simulink model "DLS_ex2"  (R2025b)
settings: Solver=VariableStepAuto  StartTime=0  StopTime=200000  FixedStep=0.5  MaxStep=200  MinStep=0.1  RelTol=.0001
model workspace (MATLAB code in the model file):
  Temp_Ambient = 295.15
  Temp_Environment = 295.15
  Time_Warmup = 200000
  Density_Copper = 8960/1000000000    (= 8.96e-06)
  Density_G10 = 1800/1000000000    (= 1.8e-06)
  Density_Stainless_Steel = 7930/1000000000    (= 7.93e-06)
  Density_Aluminium = 2700/1000000000    (= 2.7e-06)
  Density_Titanium = 4500/1000000000    (= 4.5e-06)
  Density_Aluminium_Nitride = 3300/1000000000    (= 3.3e-06)
  Density_Invar = 8050/1000000000    (= 8.05e-06)
  SHC_Copper = 386
  SHC_G10 = 500
  SHC_Stainless_Steel = 500
  SHC_Aluminium = 900
  SHC_Titanium = 528
  SHC_Aluminium_Nitride = 820
  SHC_Phosphor_Bronze = 377
  SHC_Invar = 515
  K_B1_LB = 2.83489E-08    (= 2.83489e-08)
  K_B1_RE = 1.13396E-08    (= 1.13396e-08)
  K_B1_UB = 5.66944E-09    (= 5.66944e-09)
  K_B2_LB = 5.15455E-10    (= 5.15455e-10)
  K_B2_RE = 2.3625E-10    (= 2.3625e-10)
  K_B2_UB = 9.61017E-11    (= 9.61017e-11)
  K_B3_LB = 5.15455E-09    (= 5.15455e-09)
  K_B3_RE = 2.3625E-09    (= 2.3625e-09)
  K_B3_UB = 9.61017E-10    (= 9.61017e-10)
  K_B4_LB = 5.15455E-09    (= 5.15455e-09)
  K_B4_RE = 2.3625E-09    (= 2.3625e-09)
  K_B4_UB = 9.61017E-10    (= 9.61017e-10)
  K_B5_LB = 5.15455E-09    (= 5.15455e-09)
  K_B5_RE = 2.3625E-09    (= 2.3625e-09)
  K_B5_UB = 9.61017E-10    (= 9.61017e-10)
  K_B6_LB = 5.15455E-09    (= 5.15455e-09)
  K_B6_RE = 2.3625E-09    (= 2.3625e-09)
  K_B6_UB = 9.61017E-10    (= 9.61017e-10)
  K_B7_LB = 5.67E-09    (= 5.67e-09)
  K_B7_RE = 2.8E-09    (= 2.8e-09)
  K_B7_UB = 1.11176E-09    (= 1.11176e-09)
  K_B8_LB = 5.67E-09    (= 5.67e-09)
  K_B8_RE = 2.8E-09    (= 2.8e-09)
  K_B8_UB = 1.11176E-09    (= 1.11176e-09)
  K_B9_LB = 2.835E-08    (= 2.835e-08)
  K_B9_RE = 1.08E-08    (= 1.08e-08)
  K_B9_UB = 5.15455E-09    (= 5.15455e-09)
  K_B10_LB = 4.78193E-09    (= 4.78193e-09)
  K_B10_RE = 8.95937E-10    (= 8.95937e-10)
  K_B10_UB = 2.20909E-09    (= 2.20909e-09)
  K_B13_LB = 3.54375E-09    (= 3.54375e-09)
  K_B13_RE = 1.73571E-09    (= 1.73571e-09)
  K_B13_UB = 6.85887E-10    (= 6.85887e-10)
  K_B14_LB = 2.98421E-09    (= 2.98421e-09)
  K_B14_RE = 1.45385E-09    (= 1.45385e-09)
  K_B14_UB = 5.72727E-10    (= 5.72727e-10)
  K_B15_LB = 4.05E-10    (= 4.05e-10)
  K_B15_RE = 1.95517E-10    (= 1.95517e-10)
  K_B15_UB = 5.72727E-11    (= 5.72727e-11)
  K_B16_LB = 4.05E-09    (= 4.05e-09)
  K_B16_RE = 1.95517E-09    (= 1.95517e-09)
  K_B16_UB = 5.72727E-10    (= 5.72727e-10)
  K_B17_LB = 2.83458E-09    (= 2.83458e-09)
  K_B17_RE = 1.13386E-09    (= 1.13386e-09)
  K_B17_UB = 5.66908E-10    (= 5.66908e-10)
  K_B18_LB = 2.83458E-09    (= 2.83458e-09)
  K_B18_RE = 1.13386E-09    (= 1.13386e-09)
  K_B18_UB = 5.66908E-10    (= 5.66908e-10)
  K_B19_LB = 2.83458E-09    (= 2.83458e-09)
  K_B19_RE = 1.13386E-09    (= 1.13386e-09)
  K_B19_UB = 5.66908E-10    (= 5.66908e-10)
  K_B20_LB = 5.15455E-10    (= 5.15455e-10)
  K_B20_RE = 2.3625E-10    (= 2.3625e-10)
  K_B20_UB = 9.61017E-11    (= 9.61017e-11)
  K_B21_LB = 9.45E-09    (= 9.45e-09)
  K_B21_RE = 4.05E-09    (= 4.05e-09)
  K_B21_UB = 9.61017E-10    (= 9.61017e-10)
  K_B22_LB = 4.78193E-09    (= 4.78193e-09)
  K_B22_RE = 2.20909E-09    (= 2.20909e-09)
  K_B22_UB = 8.95937E-10    (= 8.95937e-10)
  K_B23_LB = 5.15455E-09    (= 5.15455e-09)
  K_B23_RE = 2.3625E-09    (= 2.3625e-09)
  K_B23_UB = 9.61017E-10    (= 9.61017e-10)
  K_B25_LB = 2.98421E-09    (= 2.98421e-09)
  K_B25_RE = 1.45385E-09    (= 1.45385e-09)
  K_B25_UB = 5.72727E-10    (= 5.72727e-10)
  K_B1 = K_B1_RE    (= 1.13396e-08)
  K_B2 = K_B2_RE    (= 2.3625e-10)
  K_B3 = K_B3_RE    (= 2.3625e-09)
  K_B4 = K_B4_RE    (= 2.3625e-09)
  K_B5 = K_B5_RE    (= 2.3625e-09)
  K_B6 = K_B6_RE    (= 2.3625e-09)
  K_B7 = K_B7_RE    (= 2.8e-09)
  K_B8 = K_B8_RE    (= 2.8e-09)
  K_B9 = K_B9_RE    (= 1.08e-08)
  K_B10 = K_B10_RE    (= 8.95937e-10)
  K_B13 = K_B13_RE    (= 1.73571e-09)
  K_B14 = K_B14_RE    (= 1.45385e-09)
  K_B15 = K_B15_RE    (= 1.95517e-10)
  K_B16 = K_B16_RE    (= 1.95517e-09)
  K_B17 = K_B17_RE    (= 1.13386e-09)
  K_B18 = K_B18_RE    (= 1.13386e-09)
  K_B19 = K_B19_RE    (= 1.13386e-09)
  K_B20 = K_B20_RE    (= 2.3625e-10)
  K_B21 = K_B21_RE    (= 4.05e-09)
  K_B22 = K_B22_RE    (= 2.20909e-09)
  K_B23 = K_B23_RE    (= 2.3625e-09)
  K_B25 = K_B25_RE    (= 1.45385e-09)
  Area_B1 = 100000
  Area_B2 = 30000
  Area_B3 = 450
  Area_B4 = 613
  Area_B5 = 4410
  Area_B6 = 1590
  Area_B7 = 120
  Area_B8 = 50
  Area_B9 = 140
  Area_B10 = 100
  Area_B13 = 9990
  Area_B14 = 7710
  Area_B15 = 10000
  Area_B16 = 2000
  Area_B17 = 70015
  Area_B18 = 16000
  Area_B19 = 320000
  Area_B20 = 70000
  Area_B21 = 4000
  Area_B22 = 4900
  Area_B23 = 9155
  Area_B25 = 4072
  xt = linspace(5,295,2000)
  x_restemp = [4	10	20	30	40	50	60	70	80	90	100	110	120	130	140	150	160	170	180	190	200	210	220	230	240	250	260	273	280	293	300]
  y_res_A1_LB = [1.852847068	0.77281194	0.49125288	0.555353451	0.801331659	1.184325573	1.60557094	1.971748902	2.248473254	2.443766462	2.578413714	2.67150152	2.736985932	2.784247759	2.819401592	2.846406384	2.867837824	2.885389229	2.900188421	2.912997223	2.924337653	2.934572526	2.943957542	2.95267538	2.960858317	2.96860341	2.975982825	2.985117154	2.989849299	2.998335893	3.002758516]
  res_A1_LB = (akima(x_restemp,y_res_A1_LB,xt))'
  y_res_A1_RE = [1.558179157	0.649907636	0.413126378	0.467032702	0.673891715	0.995976115	1.350228639	1.658171414	1.890886853	2.055121565	2.168355165	2.246638732	2.301708818	2.34145435	2.371017486	2.393727565	2.411750652	2.426510766	2.438956365	2.449728117	2.459265019	2.467872188	2.475764655	2.48309605	2.489977612	2.496490963	2.502696791	2.51037844	2.514358008	2.521494934	2.525214205]
  res_A1_RE = (akima(x_restemp,y_res_A1_RE,xt))'
  y_res_A1_UB = [1.383495056	0.577047894	0.366811672	0.414674674	0.59834317	0.884319383	1.198857421	1.472277397	1.67890361	1.824726324	1.925265549	1.994772914	2.043669212	2.078958958	2.105207835	2.125371936	2.141374494	2.154479883	2.165530233	2.175094387	2.183562128	2.191204365	2.198212025	2.204721514	2.210831598	2.216614751	2.222124857	2.228945334	2.23247876	2.238815581	2.242117892]
  res_A1_UB = (akima(x_restemp,y_res_A1_UB,xt))'
  y_res_A2_LB = [0.466691844	0.194654505	0.123735907	0.139881445	0.201838001	0.298305832	0.40440837	0.496640627	0.566341468	0.615531576	0.649446288	0.67289308	0.689387178	0.701291403	0.710145888	0.716947808	0.722345921	0.726766738	0.730494332	0.73372059	0.736576998	0.73915494	0.741518821	0.743714655	0.745775758	0.747726578	0.749585292	0.751886031	0.753077956	0.755215544	0.756329506]
  res_A2_LB = (akima(x_restemp,y_res_A2_LB,xt))'
  y_res_A2_RE = [0.422241188	0.17611439	0.111950524	0.12655826	0.182613685	0.269893315	0.365889982	0.449337462	0.512399558	0.556904491	0.587588954	0.608802526	0.623725623	0.634496015	0.642507144	0.648661206	0.653545169	0.657544919	0.660917474	0.663836444	0.666420789	0.668753191	0.670891922	0.67287861	0.674743402	0.676508414	0.678190092	0.680271694	0.681350092	0.683284083	0.684291945]
  res_A2_RE = (akima(x_restemp,y_res_A2_RE,xt))'
  y_res_A2_UB = [0.385689258	0.160868789	0.102259362	0.115602558	0.166805463	0.246529603	0.334216178	0.410439904	0.468042936	0.508695235	0.536723452	0.55610064	0.569731897	0.579569934	0.586887568	0.592508894	0.59697007	0.600623576	0.603704181	0.606370465	0.608731093	0.610861588	0.612815176	0.614629884	0.616333247	0.617945468	0.619481569	0.621382974	0.622368019	0.624134591	0.625055206]
  res_A2_UB = (akima(x_restemp,y_res_A2_UB,xt))'
  y_res_A3_LB = [0.466691844	0.194654505	0.123735907	0.139881445	0.201838001	0.298305832	0.40440837	0.496640627	0.566341468	0.615531576	0.649446288	0.67289308	0.689387178	0.701291403	0.710145888	0.716947808	0.722345921	0.726766738	0.730494332	0.73372059	0.736576998	0.73915494	0.741518821	0.743714655	0.745775758	0.747726578	0.749585292	0.751886031	0.753077956	0.755215544	0.756329506]
  res_A3_LB = (akima(x_restemp,y_res_A3_LB,xt))'
  y_res_A3_RE = [0.422241188	0.17611439	0.111950524	0.12655826	0.182613685	0.269893315	0.365889982	0.449337462	0.512399558	0.556904491	0.587588954	0.608802526	0.623725623	0.634496015	0.642507144	0.648661206	0.653545169	0.657544919	0.660917474	0.663836444	0.666420789	0.668753191	0.670891922	0.67287861	0.674743402	0.676508414	0.678190092	0.680271694	0.681350092	0.683284083	0.684291945]
  res_A3_RE = (akima(x_restemp,y_res_A3_RE,xt))'
  y_res_A3_UB = [0.385689258	0.160868789	0.102259362	0.115602558	0.166805463	0.246529603	0.334216178	0.410439904	0.468042936	0.508695235	0.536723452	0.55610064	0.569731897	0.579569934	0.586887568	0.592508894	0.59697007	0.600623576	0.603704181	0.606370465	0.608731093	0.610861588	0.612815176	0.614629884	0.616333247	0.617945468	0.619481569	0.621382974	0.622368019	0.624134591	0.625055206]
  res_A3_UB = (akima(x_restemp,y_res_A3_UB,xt))'
  y_res_A4_LB = [1.668225823	0.695807472	0.442303498	0.500016965	0.721485431	1.066317096	1.445588764	1.77528005	2.024431055	2.200264872	2.321495613	2.405307971	2.464267391	2.506819958	2.538470996	2.562784978	2.582080948	2.597883497	2.611208069	2.622740577	2.632951025	2.642166076	2.650615951	2.658465127	2.665832701	2.672806057	2.679450173	2.68767434	2.691934966	2.699575939	2.703557883]
  res_A4_LB = (akima(x_restemp,y_res_A4_LB,xt))'
  y_res_A4_RE = [1.40291919	0.585149589	0.371961671	0.420496665	0.606743849	0.896735139	1.215689261	1.492948026	1.70247525	1.8503453	1.952296086	2.022779328	2.072362125	2.108147336	2.134764744	2.155211947	2.171439179	2.184728567	2.195934063	2.205632496	2.214219123	2.221968657	2.229074704	2.235675585	2.241871455	2.247735802	2.253323269	2.260239505	2.263822541	2.27024833	2.273597005]
  res_A4_RE = (akima(x_restemp,y_res_A4_RE,xt))'
  y_res_A4_UB = [1.245640948	0.519549732	0.330261851	0.373355692	0.538723106	0.796204099	1.079400963	1.325576846	1.511614426	1.642907084	1.733428387	1.796009905	1.840034081	1.87180749	1.895440878	1.913595789	1.928003821	1.939803364	1.949752636	1.958363799	1.965987798	1.972868548	1.979177952	1.985038822	1.990540086	1.995746994	2.000708063	2.006848934	2.010030283	2.015735691	2.018708954]
  res_A4_UB = (akima(x_restemp,y_res_A4_UB,xt))'
  y_res_A5_LB = [1.101209878	0.459308357	0.291968254	0.330065398	0.476258593	0.703884871	0.954245285	1.171877272	1.336343943	1.452413323	1.532438753	1.587763994	1.626683603	1.65477291	1.675666025	1.691715889	1.704453321	1.714884717	1.723680379	1.731293084	1.738033087	1.744116019	1.749693853	1.75487516	1.759738557	1.764341728	1.768727565	1.774156407	1.776968881	1.782012752	1.784641267]
  res_A5_LB = (akima(x_restemp,y_res_A5_LB,xt))'
  y_res_A5_RE = [0.951197386	0.396739002	0.252194832	0.285102187	0.41138019	0.607998042	0.824253069	1.012238103	1.154300276	1.254558086	1.323682039	1.37147059	1.405088369	1.429351206	1.447398153	1.461261622	1.472263895	1.481274272	1.488871744	1.495447407	1.501269252	1.506523536	1.511341528	1.515817011	1.520017891	1.523993994	1.527782369	1.532471667	1.534901011	1.53925778	1.541528225]
  res_A5_RE = (akima(x_restemp,y_res_A5_RE,xt))'
  y_res_A5_UB = [0.837873198	0.34947213	0.222148729	0.251135552	0.36236899	0.535562094	0.726052831	0.891641619	1.016778724	1.105091973	1.165980605	1.208075702	1.23768831	1.25906051	1.274957372	1.287169169	1.296860648	1.304797543	1.311489863	1.317282112	1.322410351	1.327038648	1.331282632	1.335224913	1.338925306	1.342427703	1.345764737	1.349895359	1.352035275	1.355872985	1.357872932]
  res_A5_UB = (akima(x_restemp,y_res_A5_UB,xt))'
  y_res_A6_LB = [0.466691844	0.194654505	0.123735907	0.139881445	0.201838001	0.298305832	0.40440837	0.496640627	0.566341468	0.615531576	0.649446288	0.67289308	0.689387178	0.701291403	0.710145888	0.716947808	0.722345921	0.726766738	0.730494332	0.73372059	0.736576998	0.73915494	0.741518821	0.743714655	0.745775758	0.747726578	0.749585292	0.751886031	0.753077956	0.755215544	0.756329506]
  res_A6_LB = (akima(x_restemp,y_res_A6_LB,xt))'
  y_res_A6_RE = [0.422241188	0.17611439	0.111950524	0.12655826	0.182613685	0.269893315	0.365889982	0.449337462	0.512399558	0.556904491	0.587588954	0.608802526	0.623725623	0.634496015	0.642507144	0.648661206	0.653545169	0.657544919	0.660917474	0.663836444	0.666420789	0.668753191	0.670891922	0.67287861	0.674743402	0.676508414	0.678190092	0.680271694	0.681350092	0.683284083	0.684291945]
  res_A6_RE = (akima(x_restemp,y_res_A6_RE,xt))'
  y_res_A6_UB = [0.385689258	0.160868789	0.102259362	0.115602558	0.166805463	0.246529603	0.334216178	0.410439904	0.468042936	0.508695235	0.536723452	0.55610064	0.569731897	0.579569934	0.586887568	0.592508894	0.59697007	0.600623576	0.603704181	0.606370465	0.608731093	0.610861588	0.612815176	0.614629884	0.616333247	0.617945468	0.619481569	0.621382974	0.622368019	0.624134591	0.625055206]
  res_A6_UB = (akima(x_restemp,y_res_A6_UB,xt))'
  y_res_A7_LB = [0.466691844	0.194654505	0.123735907	0.139881445	0.201838001	0.298305832	0.40440837	0.496640627	0.566341468	0.615531576	0.649446288	0.67289308	0.689387178	0.701291403	0.710145888	0.716947808	0.722345921	0.726766738	0.730494332	0.73372059	0.736576998	0.73915494	0.741518821	0.743714655	0.745775758	0.747726578	0.749585292	0.751886031	0.753077956	0.755215544	0.756329506]
  res_A7_LB = (akima(x_restemp,y_res_A7_LB,xt))'
  y_res_A7_RE = [0.422241188	0.17611439	0.111950524	0.12655826	0.182613685	0.269893315	0.365889982	0.449337462	0.512399558	0.556904491	0.587588954	0.608802526	0.623725623	0.634496015	0.642507144	0.648661206	0.653545169	0.657544919	0.660917474	0.663836444	0.666420789	0.668753191	0.670891922	0.67287861	0.674743402	0.676508414	0.678190092	0.680271694	0.681350092	0.683284083	0.684291945]
  res_A7_RE = (akima(x_restemp,y_res_A7_RE,xt))'
  y_res_A7_UB = [0.385689258	0.160868789	0.102259362	0.115602558	0.166805463	0.246529603	0.334216178	0.410439904	0.468042936	0.508695235	0.536723452	0.55610064	0.569731897	0.579569934	0.586887568	0.592508894	0.59697007	0.600623576	0.603704181	0.606370465	0.608731093	0.610861588	0.612815176	0.614629884	0.616333247	0.617945468	0.619481569	0.621382974	0.622368019	0.624134591	0.625055206]
  res_A7_UB = (akima(x_restemp,y_res_A7_UB,xt))'
  y_res_A8_LB = [2.570275206	1.072047123	0.68146752	0.770388031	1.111609765	1.642900113	2.227252994	2.735216199	3.11908908	3.390000424	3.576783511	3.705915203	3.796755384	3.862317137	3.911082643	3.948543774	3.978273534	4.002620898	4.023150383	4.040918792	4.056650273	4.070848121	4.083867043	4.095960456	4.107311852	4.118055868	4.128292615	4.140963786	4.147528232	4.159300861	4.165435938]
  res_A8_LB = (akima(x_restemp,y_res_A8_LB,xt))'
  y_res_A8_RE = [2.177935172	0.908404333	0.577444811	0.652792038	0.941927931	1.392119386	1.887273636	2.317698724	2.642975273	2.872533315	3.030804871	3.140225237	3.217199105	3.272753174	3.314074863	3.345817734	3.371009391	3.391640247	3.409036006	3.424092154	3.437422301	3.449452916	3.460484563	3.470731975	3.480350635	3.48945463	3.498128787	3.508865765	3.514428181	3.524403775	3.529602362]
  res_A8_RE = (akima(x_restemp,y_res_A8_RE,xt))'
  y_res_A8_UB = [1.891515301	0.788940239	0.501505146	0.566943472	0.818055154	1.20904201	1.639078612	2.012898573	2.29539806	2.494766965	2.632224255	2.727254769	2.794105817	2.84235398	2.878241461	2.905809833	2.927688539	2.945606235	2.960714281	2.973790398	2.985367499	2.99581597	3.005396847	3.014296624	3.022650336	3.030557066	3.038090486	3.047415446	3.052246349	3.060910055	3.065424976]
  res_A8_UB = (akima(x_restemp,y_res_A8_UB,xt))'
  y_res_A9_LB = [1.302482525	0.543258029	0.34533249	0.390392805	0.56330633	0.832536797	1.128656611	1.386066089	1.580593009	1.717876865	1.812528872	1.877966134	1.923999239	1.957222544	1.98193438	2.000917743	2.015983248	2.028321232	2.038724514	2.047728624	2.055700525	2.06289526	2.069492577	2.075620893	2.081373193	2.086817704	2.092005158	2.098426252	2.101752774	2.107718533	2.110827473]
  res_A9_LB = (akima(x_restemp,y_res_A9_LB,xt))'
  y_res_A9_RE = [1.095341951	0.456860878	0.290412467	0.328306606	0.473720793	0.700134138	0.949160477	1.165632786	1.329223078	1.444673968	1.524272974	1.579303408	1.618015628	1.645955258	1.666737042	1.682701383	1.695370942	1.705746752	1.714495546	1.722067686	1.728771774	1.734822293	1.740370404	1.745524102	1.750361583	1.754940226	1.759302692	1.764702606	1.767500094	1.772517088	1.775131596]
  res_A9_RE = (akima(x_restemp,y_res_A9_RE,xt))'
  y_res_A9_UB = [0.946128819	0.394624932	0.250850982	0.283582986	0.409188103	0.604758253	0.819860939	1.006844274	1.148149452	1.247873026	1.316628644	1.364162548	1.397601191	1.42173474	1.439685522	1.453475118	1.464418764	1.473381128	1.480938116	1.48747874	1.493269562	1.498495848	1.503288167	1.507739802	1.511918297	1.515873213	1.519641402	1.524305712	1.526722111	1.531055664	1.533314011]
  res_A9_UB = (akima(x_restemp,y_res_A9_UB,xt))'
  y_res_A10_LB = [21.77846125	8.966644519	5.100967849	4.830535038	5.997610209	8.079798747	10.41365885	12.43492555	13.94699339	15.00095825	15.71759461	16.20529908	16.54225342	16.78052084	16.95380548	17.08380935	17.18458127	17.26531026	17.33208171	17.38897845	17.43877523	17.48338116	17.52412521	17.56194268	17.59749867	17.63127075	17.6636051	17.69475498	17.72490735	17.75420153	17.78274238]
  res_A10_LB = (akima(x_restemp,y_res_A10_LB,xt))'
  y_res_A10_RE = [19.70414413	8.112605106	4.615119706	4.370444611	5.426360229	7.310228083	9.421796722	11.25054532	12.61859435	13.57217298	14.2205524	14.66180485	14.96666555	15.18223888	15.33901881	15.45664029	15.54781407	15.62085392	15.68126564	15.73274318	15.777797	15.81815438	15.85501771	15.88923321	15.92140262	15.95195804	15.98121267	16.00939564	16.03667611	16.06318013	16.08900256]
  res_A10_RE = (akima(x_restemp,y_res_A10_RE,xt))'
  y_res_A10_UB = [17.99842591	7.410325513	4.215605081	3.992110645	4.956619375	6.677407437	8.606185031	10.27662531	11.52624717	12.39727787	12.98952937	13.39258415	13.67105413	13.86796604	14.01117409	14.11861349	14.20189467	14.26861172	14.32379381	14.37081513	14.4119688	14.44883258	14.48250478	14.51375837	14.54314299	14.57105333	14.59777549	14.62351876	14.64843765	14.67264731	14.69623439]
  res_A10_UB = (akima(x_restemp,y_res_A10_UB,xt))'
  res_A11_LB = 1
  res_A11_RE = 1
  res_A11_UB = 1
  y_res_A12_LB = [0.342532347	0.142868287	0.090816994	0.102667146	0.148140674	0.218944038	0.296818875	0.364513505	0.415671015	0.451774502	0.476666486	0.493875453	0.505981433	0.514718638	0.521217461	0.526209786	0.530171776	0.533416471	0.53615237	0.538520309	0.540616793	0.542508894	0.544243885	0.545855535	0.547368299	0.54880012	0.550164338	0.551852985	0.552727807	0.554296708	0.55511431]
  res_A12_LB = (akima(x_restemp,y_res_A12_LB,xt))'
  y_res_A12_RE = [0.342532347	0.142868287	0.090816994	0.102667146	0.148140674	0.218944038	0.296818875	0.364513505	0.415671015	0.451774502	0.476666486	0.493875453	0.505981433	0.514718638	0.521217461	0.526209786	0.530171776	0.533416471	0.53615237	0.538520309	0.540616793	0.542508894	0.544243885	0.545855535	0.547368299	0.54880012	0.550164338	0.551852985	0.552727807	0.554296708	0.55511431]
  res_A12_RE = (akima(x_restemp,y_res_A12_RE,xt))'
  y_res_A12_UB = [0.342532347	0.142868287	0.090816994	0.102667146	0.148140674	0.218944038	0.296818875	0.364513505	0.415671015	0.451774502	0.476666486	0.493875453	0.505981433	0.514718638	0.521217461	0.526209786	0.530171776	0.533416471	0.53615237	0.538520309	0.540616793	0.542508894	0.544243885	0.545855535	0.547368299	0.54880012	0.550164338	0.551852985	0.552727807	0.554296708	0.55511431]
  res_A12_UB = (akima(x_restemp,y_res_A12_UB,xt))'
  res_A13_LB = 7238
  res_A13_RE = 10000
  res_A13_UB = 30000
  y_res_A14_LB = [3232.518226	329.2505618	95.9646967	56.16367989	39.40139945	30.08010454	24.15548607	20.07156297	17.09584808	14.83878298	13.07413448	11.66127195	10.50803612	9.55148427	8.747184396	8.062910655	7.474752995	6.964623057	6.518603596	6.125826366	5.777691393	5.467312659	5.189117438	4.938552014	4.711862405	4.505928832	4.318139263	4.14629174	3.988518194	3.843224457	3.709042615]
  res_A14_LB = (akima(x_restemp,y_res_A14_LB,xt))'
  y_res_A14_RE = [6244.813576	636.0701578	185.3915737	108.5010775	76.11848627	58.1109315	46.66532307	38.7757037	33.02700148	28.66663912	25.25756293	22.52809243	20.30018767	18.4522513	16.89844637	15.57651664	14.44027093	13.45476486	12.59311205	11.83431646	11.16176403	10.56215184	10.0247141	9.540653605	9.102718147	8.70488071	8.342095175	8.010107643	7.705309245	7.424620246	7.165398014]
  res_A14_RE = (akima(x_restemp,y_res_A14_RE,xt))'
  y_res_A14_UB = [55656.95959	5668.981249	1652.30414	967.0168715	678.406723	517.9142221	415.9051296	345.588823	294.3534605	255.4916901	225.1082666	200.7818351	180.9256131	164.4558628	150.6075618	138.8258506	128.6990502	119.915718	112.2362293	105.4734565	99.47932661	94.13527734	89.34535844	85.03116475	81.12806088	77.58233099	74.34900151	71.39015952	68.67364093	66.17199759	63.86167702]
  res_A14_UB = (akima(x_restemp,y_res_A14_UB,xt))'
  y_res_A15_LB = [18852.89253	1919.826452	559.4350096	327.3742072	229.6417167	175.2952947	140.7570266	116.9536284	99.61203319	86.45950823	76.17664631	67.94366255	61.22351011	55.64945847	50.96263823	46.97528904	43.54809249	40.57564411	37.97683973	35.68833978	33.66002165	31.85175061	30.23104551	28.77136414	27.4508255	26.25124518	25.1573983	24.15808684	23.237513	22.39281994	21.6098224]
  res_A15_LB = (akima(x_restemp,y_res_A15_LB,xt))'
  y_res_A15_RE = [36421.38759	3708.86023	1080.757199	632.4452798	443.6385535	338.6481869	271.9246512	225.9395169	192.4377633	167.02876	147.1635802	131.2585039	118.2760252	107.5076672	98.45332737	90.7502765	84.12936919	78.38697743	73.36641831	68.94532783	65.0268755	61.53352611	58.40253024	55.5826117	53.03149923	50.7140628	48.60088992	46.67034743	44.891916	43.26007657	41.74742503]
  res_A15_RE = (akima(x_restemp,y_res_A15_RE,xt))'
  y_res_A15_UB = [86976.01305	8856.935365	2580.899808	1510.309534	1059.430054	808.7080442	649.3690541	539.5543571	459.5505696	398.872656	351.433658	313.4515763	282.448797	256.7334439	235.1112479	216.7159945	200.9049516	187.1918459	175.2025109	164.6447357	155.2872844	146.9449992	139.4680315	132.7339314	126.6417529	121.1076041	116.0612463	111.4510186	107.2040394	103.307129	99.69484483]
  res_A15_UB = (akima(x_restemp,y_res_A15_UB,xt))'
  res_A16_LB = 3200
  res_A16_RE = 15000
  res_A16_UB = 100000
  res_A17_LB = 113.53
  res_A17_RE = 135
  res_A17_UB = 166.88
  res_A18_LB = 113.16
  res_A18_RE = 134.55
  res_A18_UB = 166.33
  res_A19_LB = 2611.7
  res_A19_RE = 2974.3
  res_A19_UB = 3458
  y_res_A20_LB = [3.730185699	1.555839171	0.988999307	1.118047753	1.613255593	2.384305966	3.232364864	3.969561053	4.526667594	4.919835462	5.19090978	5.378315857	5.510150278	5.605298654	5.676070995	5.730437537	5.773583705	5.808918516	5.838712521	5.864499435	5.887330198	5.907935233	5.926829318	5.94438023	5.960854269	5.976446831	5.991303204	6.009692605	6.019219446	6.036304812	6.045208518]
  res_A20_LB = (akima(x_restemp,y_res_A20_LB,xt))'
  y_res_A20_RE = [3.136954858	1.308405972	0.831713601	0.940238801	1.356691161	2.005117381	2.71830506	3.338261103	3.806768092	4.137408428	4.365372387	4.5229743	4.633842407	4.713858842	4.77337589	4.819096238	4.855380646	4.885095978	4.910151687	4.931837574	4.951037442	4.968365551	4.984254811	4.999014511	5.012868597	5.025981393	5.03847508	5.053939918	5.061951657	5.076319848	5.083807551]
  res_A20_RE = (akima(x_restemp,y_res_A20_RE,xt))'
  y_res_A20_UB = [2.785277622	1.161723404	0.738471985	0.834830659	1.204595444	1.780328001	2.413561749	2.964015859	3.379999541	3.673572502	3.875979914	4.015913417	4.11435234	4.185398305	4.238243025	4.278837763	4.311054405	4.337438415	4.359685183	4.378939912	4.395987324	4.411372816	4.425480766	4.438585787	4.450886722	4.462529471	4.473622518	4.487353626	4.494467186	4.50722459	4.513872863]
  res_A20_UB = (akima(x_restemp,y_res_A20_UB,xt))'
  y_res_A21_LB = [5.996914074	2.501278643	1.589986221	1.797453759	2.5935854	3.833181282	5.196581594	6.381751062	7.277395496	7.909480359	8.345278875	8.646566326	8.858512797	9.01148015	9.125258843	9.212662395	9.282027269	9.338834045	9.386733025	9.428189918	9.464894289	9.498020421	9.528395908	9.556612013	9.583096859	9.608164581	9.632048752	9.661612871	9.676928904	9.704396563	9.7187108]
  res_A21_LB = (akima(x_restemp,y_res_A21_LB,xt))'
  y_res_A21_RE = [3.802468989	1.585988119	1.00816407	1.139713208	1.644517152	2.430508888	3.295001415	4.046482942	4.614385057	5.015171705	5.291498884	5.482536503	5.616925602	5.713917757	5.78606152	5.841481574	5.885463825	5.921483351	5.951854703	5.978141314	6.001414489	6.022418808	6.041679021	6.059570034	6.076363305	6.09225802	6.107402278	6.126148027	6.135859479	6.153275924	6.162352165]
  res_A21_RE = (akima(x_restemp,y_res_A21_RE,xt))'
  y_res_A21_UB = [3.349448705	1.397035944	0.888052959	1.003929536	1.448591918	2.140941812	2.902440034	3.564391213	4.064634347	4.417671892	4.661077877	4.82935557	4.947733759	5.033170419	5.096719085	5.145536479	5.184278753	5.216006969	5.242759924	5.265914789	5.286415234	5.30491713	5.321882712	5.337642217	5.352434764	5.366435807	5.379775802	5.396288211	5.404842655	5.420184132	5.428179044]
  res_A21_UB = (akima(x_restemp,y_res_A21_UB,xt))'
  y_res_A22_LB = [0.466691844	0.194654505	0.123735907	0.139881445	0.201838001	0.298305832	0.40440837	0.496640627	0.566341468	0.615531576	0.649446288	0.67289308	0.689387178	0.701291403	0.710145888	0.716947808	0.722345921	0.726766738	0.730494332	0.73372059	0.736576998	0.73915494	0.741518821	0.743714655	0.745775758	0.747726578	0.749585292	0.751886031	0.753077956	0.755215544	0.756329506]
  res_A22_LB = (akima(x_restemp,y_res_A22_LB,xt))'
  y_res_A22_RE = [0.422241188	0.17611439	0.111950524	0.12655826	0.182613685	0.269893315	0.365889982	0.449337462	0.512399558	0.556904491	0.587588954	0.608802526	0.623725623	0.634496015	0.642507144	0.648661206	0.653545169	0.657544919	0.660917474	0.663836444	0.666420789	0.668753191	0.670891922	0.67287861	0.674743402	0.676508414	0.678190092	0.680271694	0.681350092	0.683284083	0.684291945]
  res_A22_RE = (akima(x_restemp,y_res_A22_RE,xt))'
  y_res_A22_UB = [0.385689258	0.160868789	0.102259362	0.115602558	0.166805463	0.246529603	0.334216178	0.410439904	0.468042936	0.508695235	0.536723452	0.55610064	0.569731897	0.579569934	0.586887568	0.592508894	0.59697007	0.600623576	0.603704181	0.606370465	0.608731093	0.610861588	0.612815176	0.614629884	0.616333247	0.617945468	0.619481569	0.621382974	0.622368019	0.624134591	0.625055206]
  res_A22_UB = (akima(x_restemp,y_res_A22_UB,xt))'
  y_res_A23_LB = [0.466691844	0.194654505	0.123735907	0.139881445	0.201838001	0.298305832	0.40440837	0.496640627	0.566341468	0.615531576	0.649446288	0.67289308	0.689387178	0.701291403	0.710145888	0.716947808	0.722345921	0.726766738	0.730494332	0.73372059	0.736576998	0.73915494	0.741518821	0.743714655	0.745775758	0.747726578	0.749585292	0.751886031	0.753077956	0.755215544	0.756329506]
  res_A23_LB = (akima(x_restemp,y_res_A23_LB,xt))'
  y_res_A23_RE = [0.422241188	0.17611439	0.111950524	0.12655826	0.182613685	0.269893315	0.365889982	0.449337462	0.512399558	0.556904491	0.587588954	0.608802526	0.623725623	0.634496015	0.642507144	0.648661206	0.653545169	0.657544919	0.660917474	0.663836444	0.666420789	0.668753191	0.670891922	0.67287861	0.674743402	0.676508414	0.678190092	0.680271694	0.681350092	0.683284083	0.684291945]
  res_A23_RE = (akima(x_restemp,y_res_A23_RE,xt))'
  y_res_A23_UB = [0.385689258	0.160868789	0.102259362	0.115602558	0.166805463	0.246529603	0.334216178	0.410439904	0.468042936	0.508695235	0.536723452	0.55610064	0.569731897	0.579569934	0.586887568	0.592508894	0.59697007	0.600623576	0.603704181	0.606370465	0.608731093	0.610861588	0.612815176	0.614629884	0.616333247	0.617945468	0.619481569	0.621382974	0.622368019	0.624134591	0.625055206]
  res_A23_UB = (akima(x_restemp,y_res_A23_UB,xt))'
  y_res_A24_LB = [5.996914074	2.501278643	1.589986221	1.797453759	2.5935854	3.833181282	5.196581594	6.381751062	7.277395496	7.909480359	8.345278875	8.646566326	8.858512797	9.01148015	9.125258843	9.212662395	9.282027269	9.338834045	9.386733025	9.428189918	9.464894289	9.498020421	9.528395908	9.556612013	9.583096859	9.608164581	9.632048752	9.661612871	9.676928904	9.704396563	9.7187108]
  res_A24_LB = (akima(x_restemp,y_res_A24_LB,xt))'
  y_res_A24_RE = [3.802468989	1.585988119	1.00816407	1.139713208	1.644517152	2.430508888	3.295001415	4.046482942	4.614385057	5.015171705	5.291498884	5.482536503	5.616925602	5.713917757	5.78606152	5.841481574	5.885463825	5.921483351	5.951854703	5.978141314	6.001414489	6.022418808	6.041679021	6.059570034	6.076363305	6.09225802	6.107402278	6.126148027	6.135859479	6.153275924	6.162352165]
  res_A24_RE = (akima(x_restemp,y_res_A24_RE,xt))'
  y_res_A24_UB = [3.349448705	1.397035944	0.888052959	1.003929536	1.448591918	2.140941812	2.902440034	3.564391213	4.064634347	4.417671892	4.661077877	4.82935557	4.947733759	5.033170419	5.096719085	5.145536479	5.184278753	5.216006969	5.242759924	5.265914789	5.286415234	5.30491713	5.321882712	5.337642217	5.352434764	5.366435807	5.379775802	5.396288211	5.404842655	5.420184132	5.428179044]
  res_A24_UB = (akima(x_restemp,y_res_A24_UB,xt))'
  y_res_A25_LB = [3.385783654	1.412191043	0.897686592	1.014820202	1.464306299	2.164166831	2.933925815	3.603057866	4.108727656	4.465594967	4.711641429	4.881744604	5.001406965	5.087770445	5.15200849	5.201355456	5.240518008	5.272590412	5.299633585	5.323039635	5.34376247	5.362465075	5.3796147	5.395545165	5.410498182	5.424651108	5.438135816	5.454827352	5.463474596	5.478982497	5.487064139]
  res_A25_LB = (akima(x_restemp,y_res_A25_LB,xt))'
  y_res_A25_RE = [2.91220524	1.214664189	0.772124821	0.872874647	1.259489947	1.861459157	2.523549939	3.09908874	3.534029174	3.840980521	4.052611821	4.198922221	4.301847094	4.376130688	4.431383589	4.473828267	4.50751305	4.535099403	4.558359977	4.578492161	4.596316439	4.612403062	4.627153924	4.640856153	4.653717652	4.665890972	4.677489539	4.691846386	4.699284117	4.712622888	4.719574129]
  res_A25_RE = (akima(x_restemp,y_res_A25_RE,xt))'
  y_res_A25_UB = [2.557152629	1.066573771	0.677988278	0.766454804	1.105934426	1.634512263	2.215881721	2.721251514	3.103164526	3.372692728	3.558522191	3.6869946	3.777370995	3.842598021	3.891114554	3.928384427	3.957962401	3.982185459	4.002610131	4.020287823	4.035938986	4.050064347	4.063016801	4.075048471	4.086341912	4.097031075	4.107215558	4.119822035	4.126352967	4.138065491	4.144169244]
  res_A25_UB = (akima(x_restemp,y_res_A25_UB,xt))'
  y_res_A26_LB = [0.466691844	0.194654505	0.123735907	0.139881445	0.201838001	0.298305832	0.40440837	0.496640627	0.566341468	0.615531576	0.649446288	0.67289308	0.689387178	0.701291403	0.710145888	0.716947808	0.722345921	0.726766738	0.730494332	0.73372059	0.736576998	0.73915494	0.741518821	0.743714655	0.745775758	0.747726578	0.749585292	0.751886031	0.753077956	0.755215544	0.756329506]
  res_A26_LB = (akima(x_restemp,y_res_A26_LB,xt))'
  y_res_A26_RE = [0.422241188	0.17611439	0.111950524	0.12655826	0.182613685	0.269893315	0.365889982	0.449337462	0.512399558	0.556904491	0.587588954	0.608802526	0.623725623	0.634496015	0.642507144	0.648661206	0.653545169	0.657544919	0.660917474	0.663836444	0.666420789	0.668753191	0.670891922	0.67287861	0.674743402	0.676508414	0.678190092	0.680271694	0.681350092	0.683284083	0.684291945]
  res_A26_RE = (akima(x_restemp,y_res_A26_RE,xt))'
  y_res_A26_UB = [0.385689258	0.160868789	0.102259362	0.115602558	0.166805463	0.246529603	0.334216178	0.410439904	0.468042936	0.508695235	0.536723452	0.55610064	0.569731897	0.579569934	0.586887568	0.592508894	0.59697007	0.600623576	0.603704181	0.606370465	0.608731093	0.610861588	0.612815176	0.614629884	0.616333247	0.617945468	0.619481569	0.621382974	0.622368019	0.624134591	0.625055206]
  res_A26_UB = (akima(x_restemp,y_res_A26_UB,xt))'
  y_res_A27_LB = [0.466691844	0.194654505	0.123735907	0.139881445	0.201838001	0.298305832	0.40440837	0.496640627	0.566341468	0.615531576	0.649446288	0.67289308	0.689387178	0.701291403	0.710145888	0.716947808	0.722345921	0.726766738	0.730494332	0.73372059	0.736576998	0.73915494	0.741518821	0.743714655	0.745775758	0.747726578	0.749585292	0.751886031	0.753077956	0.755215544	0.756329506]
  res_A27_LB = (akima(x_restemp,y_res_A27_LB,xt))'
  y_res_A27_RE = [0.422241188	0.17611439	0.111950524	0.12655826	0.182613685	0.269893315	0.365889982	0.449337462	0.512399558	0.556904491	0.587588954	0.608802526	0.623725623	0.634496015	0.642507144	0.648661206	0.653545169	0.657544919	0.660917474	0.663836444	0.666420789	0.668753191	0.670891922	0.67287861	0.674743402	0.676508414	0.678190092	0.680271694	0.681350092	0.683284083	0.684291945]
  res_A27_RE = (akima(x_restemp,y_res_A27_RE,xt))'
  y_res_A27_UB = [0.385689258	0.160868789	0.102259362	0.115602558	0.166805463	0.246529603	0.334216178	0.410439904	0.468042936	0.508695235	0.536723452	0.55610064	0.569731897	0.579569934	0.586887568	0.592508894	0.59697007	0.600623576	0.603704181	0.606370465	0.608731093	0.610861588	0.612815176	0.614629884	0.616333247	0.617945468	0.619481569	0.621382974	0.622368019	0.624134591	0.625055206]
  res_A27_UB = (akima(x_restemp,y_res_A27_UB,xt))'
  y_res_A28_LB = [3.385783654	1.412191043	0.897686592	1.014820202	1.464306299	2.164166831	2.933925815	3.603057866	4.108727656	4.465594967	4.711641429	4.881744604	5.001406965	5.087770445	5.15200849	5.201355456	5.240518008	5.272590412	5.299633585	5.323039635	5.34376247	5.362465075	5.3796147	5.395545165	5.410498182	5.424651108	5.438135816	5.454827352	5.463474596	5.478982497	5.487064139]
  res_A28_LB = (akima(x_restemp,y_res_A28_LB,xt))'
  y_res_A28_RE = [2.91220524	1.214664189	0.772124821	0.872874647	1.259489947	1.861459157	2.523549939	3.09908874	3.534029174	3.840980521	4.052611821	4.198922221	4.301847094	4.376130688	4.431383589	4.473828267	4.50751305	4.535099403	4.558359977	4.578492161	4.596316439	4.612403062	4.627153924	4.640856153	4.653717652	4.665890972	4.677489539	4.691846386	4.699284117	4.712622888	4.719574129]
  res_A28_RE = (akima(x_restemp,y_res_A28_RE,xt))'
  y_res_A28_UB = [2.557152629	1.066573771	0.677988278	0.766454804	1.105934426	1.634512263	2.215881721	2.721251514	3.103164526	3.372692728	3.558522191	3.6869946	3.777370995	3.842598021	3.891114554	3.928384427	3.957962401	3.982185459	4.002610131	4.020287823	4.035938986	4.050064347	4.063016801	4.075048471	4.086341912	4.097031075	4.107215558	4.119822035	4.126352967	4.138065491	4.144169244]
  res_A28_UB = (akima(x_restemp,y_res_A28_UB,xt))'
  res_A31_LB = 113.53
  res_A31_RE = 135
  res_A31_UB = 166.88
  res_A32_LB = 113.53
  res_A32_RE = 135
  res_A32_UB = 166.88
  res_A33_LB = 113.53
  res_A33_RE = 135
  res_A33_UB = 166.88
  res_A34_LB = 106.89
  res_A34_RE = 127.1
  res_A34_UB = 157.12
  res_A36_LB = 100
  res_A36_RE = 100
  res_A36_UB = 100
  y_res_A37_LB = [559.0264465	277.2362191	143.0749777	104.5075798	87.00904569	78.13471948	71.71197015	67.96291148	65.29305409	62.842993	60.67239457	58.91033361	57.3420793	55.60751686	53.98751593	52.67332244	51.36613692	50.09621037	48.99723247	48.01630621	46.85892867	45.6703913	44.78832759	44.04526831	43.31563014	42.56138686	41.81566865	40.7882804	40.20917218	39.33052889	38.95803316]
  res_A37_LB = (akima(x_restemp,y_res_A37_LB,xt))'
  y_res_A37_RE = [647.1900089	320.958896	165.6392048	120.9893771	100.7311647	90.45727643	83.02160102	78.68128165	75.59036344	72.75390539	70.24098382	68.20102979	66.38544749	64.37732876	62.50183893	60.98038516	59.46704457	57.99683904	56.72454231	55.58891505	54.24900852	52.87302799	51.8518548	50.9916083	50.14689955	49.27370523	48.41038047	47.22096373	46.55052488	45.53331153	45.10206983]
  res_A37_RE = (akima(x_restemp,y_res_A37_RE,xt))'
  y_res_A37_UB = [769.5803815	381.6555667	196.963304	143.8697286	119.7804773	107.5636897	98.72185062	93.56073165	89.8852886	86.51242679	83.52428557	81.09855499	78.93962716	76.55175226	74.32158777	72.51241124	70.71288218	68.96464546	67.45174417	66.10135796	64.50806116	62.87186837	61.6575807	60.63465262	59.63020065	58.59187618	57.56528771	56.15093988	55.35371406	54.14413507	53.63134107]
  ... (+210 more variables)
libraries: fl_lib x606, nesl_utility x187, slpidlib x8, simulink x2
(part 13 of 17)

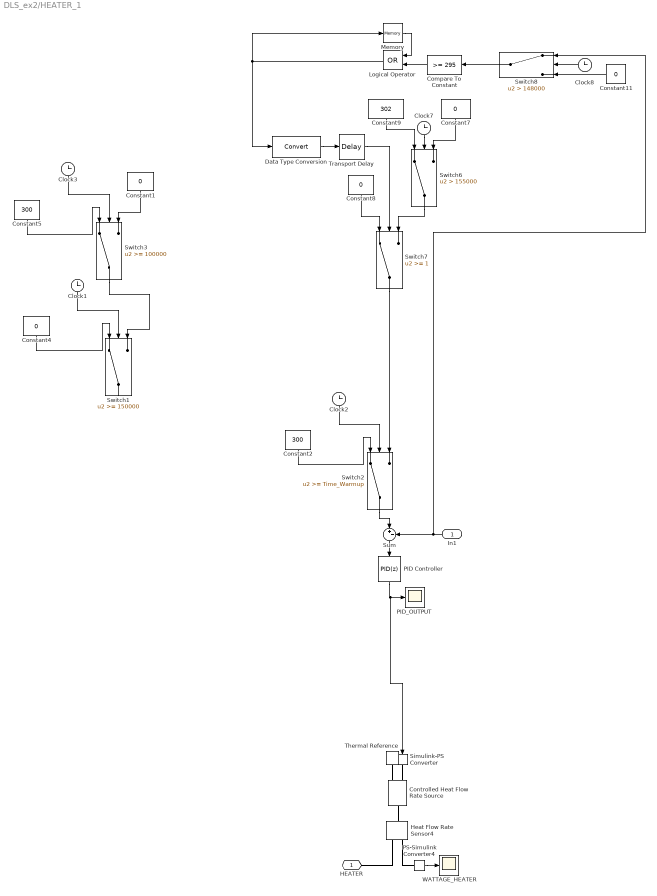
== system DLS_ex2/HEATER_1 ==
  In1 : Inport
  Clock{1..3,7..8} (5 alike) : Clock
  Compare To Constant : simulink/Logic and Bit Operations/Compare To Constant  relop=>=  const=295  OutDataTypeStr=boolean
  Constant{1,4,7..8,11} (5 alike) : Constant  Value=0
  Constant2 : Constant  Value=300
  Constant5 : Constant  Value=300
  Constant9 : Constant  Value=302
  Controlled Heat Flow Rate Source : fl_lib/Thermal/Thermal Sources/Controlled Heat Flow Rate Source
  Data Type Conversion : DataTypeConversion  SaturateOnIntegerOverflow=off  RndMeth=Floor
  Heat Flow Rate Sensor4 : fl_lib/Thermal/Thermal Sensors/Heat Flow Rate Sensor
  Logical Operator : Logic  Operator=OR  AllPortsSameDT=off
  Memory : Memory  LinearizeMemory=on  LinearizeAsDelay=on
  PID Controller : slpidlib/PID Controller  Controller=PID  Form=Parallel  TimeDomain=Discrete-time  UseExternalTs=off  SampleTime=-1  IntegratorMethod=Forward Euler  FilterMethod=Forward Euler  ControllerParametersSource=internal  P=10  I=0.001  UseKiTs=off  D=0  UseExternalDerivativeSource=off  N=100  UseFilter=on  TunerSelectOption=Transfer Function Based (PID Tuner App)  ZeroCross=off  InitialConditionSource=internal  InitialConditionForIntegrator=0  InitialConditionForFilter=0  DifferentiatorICPrevScaledInput=0  ExternalReset=none  TrackingMode=off  Kt=1  LimitOutput=on  SatLimitsSource=internal  UpperSaturationLimit=20  LowerSaturationLimit=0  LinearizeAsGain=on  AntiWindupMode=clamping  Kb=1  LimitIntegrator=off  UpperIntegratorSaturationLimit=inf  LowerIntegratorSaturationLimit=-inf  POutMin=[]  POutMax=[]  IOutMin=[]  IOutMax=[]  DOutMin=[]  DOutMax=[]  NOutMin=[]  NOutMax=[]  SumOutMin=[]  SumOutMax=[]  SaturationOutMin=[]  SaturationOutMax=[]  PParamMin=[]  PParamMax=[]  IParamMin=[]  IParamMax=[]  DParamMin=[]  DParamMax=[]  NParamMin=[]  NParamMax=[]  KbParamMin=[]  KbParamMax=[]  KtParamMin=[]  KtParamMax=[]  KbOutMin=[]  KbOutMax=[]  KtOutMin=[]  KtOutMax=[]  IntegratorOutMin=[]  IntegratorOutMax=[]  FilterOutMin=[]  FilterOutMax=[]  SumI1OutMin=[]  SumI1OutMax=[]  SumI2OutMin=[]  SumI2OutMax=[]  SumI3OutMin=[]  SumI3OutMax=[]  SumI4OutMin=[]  SumI4OutMax=[]  SumDOutMin=[]  SumDOutMax=[]  DifferentiatorOutMin=[]  DifferentiatorOutMax=[]  FilterDiffOutCoefMin=[]  FilterDiffOutCoefMax=[]  ReciprocalOutMin=[]  ReciprocalOutMax=[]  SumDenOutMin=[]  SumDenOutMax=[]  SumNumOutMin=[]  SumNumOutMax=[]  DivideOutMin=[]  DivideOutMax=[]  UdiffTsProdOutMin=[]  UdiffTsProdOutMax=[]  NTsProdOutMin=[]  NTsProdOutMax=[]  UintegralTsProdOutMin=[]  UintegralTsProdOutMax=[]  UngainTsProdOutMin=[]  UngainTsProdOutMax=[]  ClampingZeroOutDataTypeStr=Inherit: Inherit via back propagation  ClampingZeroOutMin=[]  ClampingZeroOutMax=[]  FilterDenConstantOutDataTypeStr=Inherit: Inherit via back propagation  FilterDenConstantOutMin=[]  FilterDenConstantOutMax=[]  PCopyOutDataTypeStr=Inherit: Inherit via back propagation  PCopyOutMin=[]  PCopyOutMax=[]  NCopyOutDataTypeStr=Inherit: Inherit via back propagation  NCopyOutMin=[]  NCopyOutMax=[]  IntegratorContinuousStateAttributes=''  IntegratorStateMustResolveToSignalObject=off  IntegratorRTWStateStorageClass=Auto  FilterContinuousStateAttributes=''  FilterStateMustResolveToSignalObject=off  FilterRTWStateStorageClass=Auto  ParallelPVariant=InternalParameters  IdealPVariant=Disabled  IVariant=InternalParameters  DVariant=InternalParameters  IntegratorVariant=Discrete  SatVariant=Enabled  AWVariant=DiscClampingParallel  PCopyVariant=Disabled  TRVariant=Disabled  FdbkBlocksVariant=Forward  IdealPFdbkVariant=Disabled  SatFdbkVariant=Disabled  DerivativeFilterVariant=ForwardEulerFilter  NVariant=InternalParameters  NCopyVariant=Disabled  FilterICVariant=InternalICsFilter  IntegratorICVariant=InternalICs  ExternalResetVariant=Disabled  TRSumVariant=Passthrough  SumFdbkVariant=Disabled  SumVariant=Sum_PID  TsampFilterVariant=InternalTs  TsampNgainVariant=Passthrough  TsampIntegralVariant=Disabled_SignalSpec  ExternalSaturationOutDataTypeStr=Inherit: Same as second input  DerivativeSourceVariant=ErrorSignal  PreIntVariant=InternalPreInt
  PID_OUTPUT : Scope
      settings: ActiveDisplayYMinimum=-6.25  ActiveDisplayYMaximum=56.25
  PS-Simulink Converter4 : nesl_utility/PS-Simulink Converter  PhysicalDomain=network_engine_domain  SubClassName=ps_output  LeftPortType=input  RightPortType=output  PseudoPeriodic=off  Frequencies=[]  VectorFormat=inherit  Unit=inherit  AffineConversion=off
  Simulink-PS Converter : nesl_utility/Simulink-PS Converter  PhysicalDomain=network_engine_domain  SubClassName=ps_input  LeftPortType=input  RightPortType=output  PseudoPeriodic=off  Frequencies=[]  NoiseDistribution=none  NoiseParameters=[]  Unit=1  AffineConversion=off  FilteringAndDerivatives=provide  SimscapeFilterOrder=1  InputFilterTimeConstant=0.001  UdotUserProvided=0
  Sum : Sum  Inputs=|+-
  Switch1 : Switch  Threshold=150000  SaturateOnIntegerOverflow=off  InputSameDT=off
  Switch2 : Switch  Threshold=Time_Warmup  SaturateOnIntegerOverflow=off  InputSameDT=off
  Switch3 : Switch  Threshold=100000  SaturateOnIntegerOverflow=off  InputSameDT=off
  Switch6 : Switch  Criteria=u2 > Threshold  Threshold=155000  SaturateOnIntegerOverflow=off  InputSameDT=off
  Switch7 : Switch  Threshold=1  SaturateOnIntegerOverflow=off  InputSameDT=off
  Switch8 : Switch  Criteria=u2 > Threshold  Threshold=148000  ZeroCross=off  SaturateOnIntegerOverflow=off  InputSameDT=off
  Thermal Reference : fl_lib/Thermal/Thermal Elements/Thermal Reference
  Transport Delay : TransportDelay  DelayTime=60
  WATTAGE_HEATER : Scope
      settings: ActiveDisplayYMinimum=-6.25  ActiveDisplayYMaximum=56.25  DataLoggingVariableName=ScopeData3
  HEATER : PMIOPort  Side=Right
  wires:
  PS-Simulink Converter4/1 -> WATTAGE_HEATER/1
  Sum/1 -> PID Controller/1
  Clock7/1 -> Switch6/2
  Constant9/1 -> Switch6/1
  Constant7/1 -> Switch6/3
  Constant8/1 -> Switch7/1
  Switch6/1 -> Switch7/3
  PID Controller/1 -> Simulink-PS Converter/1, PID_OUTPUT/1
  In1/1 -> Sum/2, Switch8/1
  Constant11/1 -> Switch8/3
  Clock8/1 -> Switch8/2
  Compare To Constant/1 -> Logical Operator/2
  Switch8/1 -> Compare To Constant/1
  Memory/1 -> Logical Operator/1
  Logical Operator/1 -> Memory/1, Data Type Conversion/1
  Transport Delay/1 -> Switch7/2
  Data Type Conversion/1 -> Transport Delay/1
  Constant2/1 -> Switch2/1
  Clock2/1 -> Switch2/2
  Switch2/1 -> Sum/1
  Switch3/1 -> Switch1/3
  Constant4/1 -> Switch1/1
  Clock1/1 -> Switch1/2
  Clock3/1 -> Switch3/2
  Constant1/1 -> Switch3/3
  Constant5/1 -> Switch3/1
  Switch7/1 -> Switch2/3
  connections:
  Heat Flow Rate Sensor4/RConn2 -- HEATER/RConn1
  Thermal Reference/LConn1 -- Controlled Heat Flow Rate Source/RConn2
  Heat Flow Rate Sensor4/RConn1 -- PS-Simulink Converter4/LConn1
  Controlled Heat Flow Rate Source/LConn1 -- Heat Flow Rate Sensor4/LConn1
  Simulink-PS Converter/RConn1 -- Controlled Heat Flow Rate Source/RConn1

== system DLS_ex2/HEATER_2 ==
  In1 : Inport
  1-D Lookup Table : Lookup_n-D  Commented=on  NumberOfTableDimensions=1  BreakpointsForDimension1=xt  Table=WATTAGE_HEATER  InternalRulePriority=Speed  RndMeth=Simplest
  Clock4 : Clock  Commented=on
  Clock7 : Clock  Commented=on
  Constant10 : Constant  Value=300
  Constant2 : Constant  Commented=on  Value=0
  Controlled Heat Flow Rate Source : fl_lib/Thermal/Thermal Sources/Controlled Heat Flow Rate Source
  Fcn : Fcn  Commented=on  Expr=-(50/2000)*(u-75000)
  Heat Flow Rate Sensor4 : fl_lib/Thermal/Thermal Sensors/Heat Flow Rate Sensor
  PID Controller : slpidlib/PID Controller  Controller=PID  Form=Parallel  TimeDomain=Discrete-time  UseExternalTs=off  SampleTime=-1  IntegratorMethod=Forward Euler  FilterMethod=Forward Euler  ControllerParametersSource=internal  P=10  I=0.001  UseKiTs=off  D=0  UseExternalDerivativeSource=off  N=100  UseFilter=on  TunerSelectOption=Transfer Function Based (PID Tuner App)  InitialConditionSource=internal  InitialConditionForIntegrator=0  InitialConditionForFilter=0  DifferentiatorICPrevScaledInput=0  ExternalReset=none  TrackingMode=off  Kt=1  LimitOutput=on  SatLimitsSource=internal  UpperSaturationLimit=50  LowerSaturationLimit=0  LinearizeAsGain=on  AntiWindupMode=clamping  Kb=1  LimitIntegrator=off  UpperIntegratorSaturationLimit=inf  LowerIntegratorSaturationLimit=-inf  POutMin=[]  POutMax=[]  IOutMin=[]  IOutMax=[]  DOutMin=[]  DOutMax=[]  NOutMin=[]  NOutMax=[]  SumOutMin=[]  SumOutMax=[]  SaturationOutMin=[]  SaturationOutMax=[]  PParamMin=[]  PParamMax=[]  IParamMin=[]  IParamMax=[]  DParamMin=[]  DParamMax=[]  NParamMin=[]  NParamMax=[]  KbParamMin=[]  KbParamMax=[]  KtParamMin=[]  KtParamMax=[]  KbOutMin=[]  KbOutMax=[]  KtOutMin=[]  KtOutMax=[]  IntegratorOutMin=[]  IntegratorOutMax=[]  FilterOutMin=[]  FilterOutMax=[]  SumI1OutMin=[]  SumI1OutMax=[]  SumI2OutMin=[]  SumI2OutMax=[]  SumI3OutMin=[]  SumI3OutMax=[]  SumI4OutMin=[]  SumI4OutMax=[]  SumDOutMin=[]  SumDOutMax=[]  DifferentiatorOutMin=[]  DifferentiatorOutMax=[]  FilterDiffOutCoefMin=[]  FilterDiffOutCoefMax=[]  ReciprocalOutMin=[]  ReciprocalOutMax=[]  SumDenOutMin=[]  SumDenOutMax=[]  SumNumOutMin=[]  SumNumOutMax=[]  DivideOutMin=[]  DivideOutMax=[]  UdiffTsProdOutMin=[]  UdiffTsProdOutMax=[]  NTsProdOutMin=[]  NTsProdOutMax=[]  UintegralTsProdOutMin=[]  UintegralTsProdOutMax=[]  UngainTsProdOutMin=[]  UngainTsProdOutMax=[]  ClampingZeroOutDataTypeStr=Inherit: Inherit via back propagation  ClampingZeroOutMin=[]  ClampingZeroOutMax=[]  FilterDenConstantOutDataTypeStr=Inherit: Inherit via back propagation  FilterDenConstantOutMin=[]  FilterDenConstantOutMax=[]  PCopyOutDataTypeStr=Inherit: Inherit via back propagation  PCopyOutMin=[]  PCopyOutMax=[]  NCopyOutDataTypeStr=Inherit: Inherit via back propagation  NCopyOutMin=[]  NCopyOutMax=[]  IntegratorContinuousStateAttributes=''  IntegratorStateMustResolveToSignalObject=off  IntegratorRTWStateStorageClass=Auto  FilterContinuousStateAttributes=''  FilterStateMustResolveToSignalObject=off  FilterRTWStateStorageClass=Auto  ParallelPVariant=InternalParameters  IdealPVariant=Disabled  IVariant=InternalParameters  DVariant=InternalParameters  IntegratorVariant=Discrete  SatVariant=Enabled  AWVariant=DiscClampingParallel  PCopyVariant=Disabled  TRVariant=Disabled  FdbkBlocksVariant=Forward  IdealPFdbkVariant=Disabled  SatFdbkVariant=Disabled  DerivativeFilterVariant=ForwardEulerFilter  NVariant=InternalParameters  NCopyVariant=Disabled  FilterICVariant=InternalICsFilter  IntegratorICVariant=InternalICs  ExternalResetVariant=Disabled  TRSumVariant=Passthrough  SumFdbkVariant=Disabled  SumVariant=Sum_PID  TsampFilterVariant=InternalTs  TsampNgainVariant=Passthrough  TsampIntegralVariant=Disabled_SignalSpec  ExternalSaturationOutDataTypeStr=Inherit: Same as second input  DerivativeSourceVariant=ErrorSignal  PreIntVariant=InternalPreInt
  PID_OUTPUT : Scope
      settings: ActiveDisplayYMinimum=-6.05668  ActiveDisplayYMaximum=56.22852  DataLoggingVariableName=ScopeData3
  PS-Simulink Converter4 : nesl_utility/PS-Simulink Converter  PhysicalDomain=network_engine_domain  SubClassName=ps_output  LeftPortType=input  RightPortType=output  PseudoPeriodic=off  Frequencies=[]  VectorFormat=inherit  Unit=inherit  AffineConversion=off
  Simulink-PS Converter : nesl_utility/Simulink-PS Converter  PhysicalDomain=network_engine_domain  SubClassName=ps_input  LeftPortType=input  RightPortType=output  PseudoPeriodic=off  Frequencies=[]  NoiseDistribution=none  NoiseParameters=[]  Unit=1  AffineConversion=off  FilteringAndDerivatives=provide  SimscapeFilterOrder=1  InputFilterTimeConstant=0.001  UdotUserProvided=0
  Sum : Sum  Inputs=|+-
  Switch4 : Switch  Commented=on  Criteria=u2 > Threshold  SaturateOnIntegerOverflow=off  InputSameDT=off
  Thermal Reference : fl_lib/Thermal/Thermal Elements/Thermal Reference
  WATTAGE_HEATER : Scope
      settings: ActiveDisplayYMinimum=-6.05664  ActiveDisplayYMaximum=56.22852  DataLoggingVariableName=ScopeData3
  HEATER : PMIOPort  Side=Right
  wires:
  PS-Simulink Converter4/1 -> WATTAGE_HEATER/1
  Clock7/1 -> Fcn/1
  Clock4/1 -> Switch4/2
  1-D Lookup Table/1 -> Switch4/1
  Constant2/1 -> Switch4/3
  PID Controller/1 -> Simulink-PS Converter/1, PID_OUTPUT/1
  Constant10/1 -> Sum/1
  Sum/1 -> PID Controller/1
  In1/1 -> Sum/2
  connections:
  Heat Flow Rate Sensor4/RConn2 -- HEATER/RConn1
  Thermal Reference/LConn1 -- Controlled Heat Flow Rate Source/RConn2
  Heat Flow Rate Sensor4/RConn1 -- PS-Simulink Converter4/LConn1
  Controlled Heat Flow Rate Source/LConn1 -- Heat Flow Rate Sensor4/LConn1
  Simulink-PS Converter/RConn1 -- Controlled Heat Flow Rate Source/RConn1
